simulink model "V2L"  (R2023a)
settings: Solver=ode23t  StartTime=0.0  StopTime=1  MaxStep=1e-4  RelTol=1e-3
undefined symbols (not defined in the file): Ion, Lithium
libraries: spsSeriesRLCBranchLib x5, spsCurrentMeasurementLib x2, spsVoltageMeasurementLib x2, spsBatteryLib x1, spsDiodeLib x1, spsMosfetLib x1, spsSeriesRLCLoadLib x1, slpidlib x1, spsPWMGenerator2LevelLib x1, spsPWMGeneratorDCDCLib x1, spsUniversalBridgeLib x1, spspowerguiLib x1
settings Model: Creator=Alielden  LastModifiedBy=Alielden

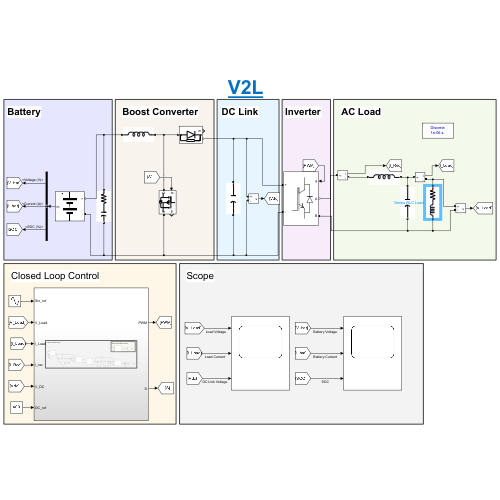
[thumbnail: Simulink's stored preview of the top-level diagram]
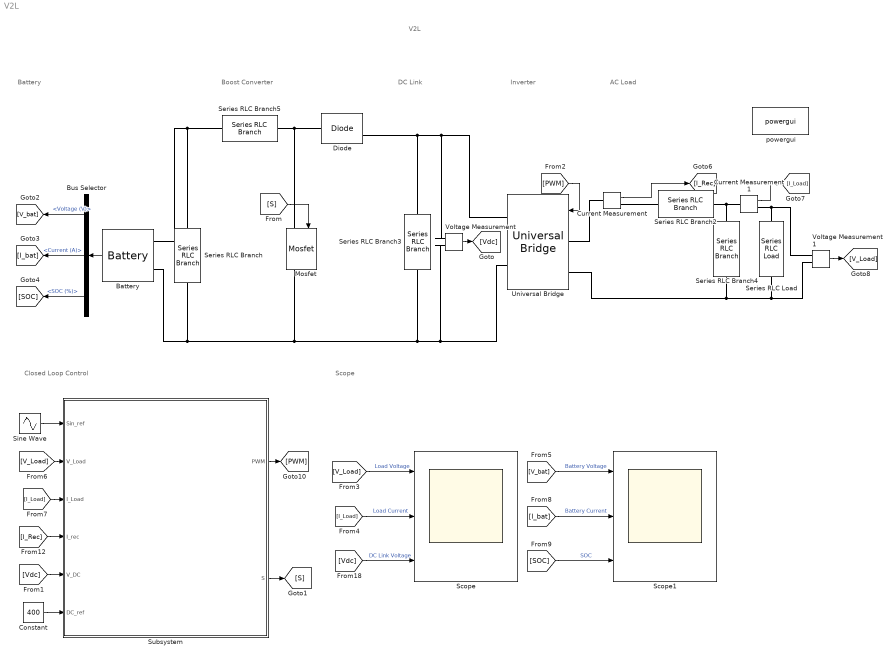
== system V2L ==
  note: Battery
  note: Boost Converter
  note: DC Link
  note: Inverter
  note: AC Load
  note: Closed Loop Control
  note: Scope
  note: V2L
  Battery : spsBatteryLib/Battery  BatType=Lithium-Ion  ShowTempParam=off  ThermalPreset=no  ShowAgeParam=off  NomV=160  NomQ=120  SOC=50  Batt_Tr=1  PresetModel=on  MaxQ=120  MinV=120  FullV=186.2379  Dis_rate=52.1739  R=0.013333  Normal_OP=108.5217  expZone="[172.8617      5.895652]"  current=[6.5 13 32.5]  Units=Time  Tci=20  NomT=20  T2=-30  MaxQ2=4.8  FullV2=7.1  Normal_OP2=5.655  expZone2="[6.58           1]"  Rca=0.6  ti=2000  Dp=0  Neq0=0  Tsim=1e6  Ta1=25  Qeol=5.4*0.9  Reol=0.013333*1.2  Char_age=[2.3478, 3]  Dis_age=[2.3478, 10]  N1=1500  N2=10500  N3=1000  N4=1400  Ta2=45  N5=950
  Bus Selector : BusSelector  OutputSignals=Voltage (V),Current (A),SOC (%)
  Constant : Constant  Value=400
  Current Measurement : spsCurrentMeasurementLib/Current Measurement  PhasorSimulation=off  OutputType=Complex  PSBequivalent=0
  Current Measurement1 : spsCurrentMeasurementLib/Current Measurement  PhasorSimulation=off  OutputType=Complex  PSBequivalent=0
  Diode : spsDiodeLib/Diode  Ron=0.001  Lon=0  Vf=0.8  IC=0  UseSnubber=0  Rs=500  Cs=250e-9  Measurements=on
  Mosfet : spsMosfetLib/Mosfet  Ron=0.1  Lon=0  Rd=0.01  Vfd=0  IC=0  Rs=1e5  Cs=inf  Measurements=on
  Scope : Scope  NumInputPorts=3
  Scope1 : Scope  NumInputPorts=3
  Series RLC Branch : spsSeriesRLCBranchLib/Series RLC Branch  LConnTagsString=__new0  RConnTagsString=__new0  BranchType=RC  Resistance=0.0001  Inductance=1e-3  SetiL0=off  InitialCurrent=0  Capacitance=100e-6  Setx0=off  InitialVoltage=0  Measurements=None
  Series RLC Branch2 : spsSeriesRLCBranchLib/Series RLC Branch  LConnTagsString=__new0  RConnTagsString=__new0  BranchType=L  Resistance=1  Inductance=2e-3  SetiL0=off  InitialCurrent=0  Capacitance=5600e-6  Setx0=off  InitialVoltage=400  Measurements=None
  Series RLC Branch3 : spsSeriesRLCBranchLib/Series RLC Branch  LConnTagsString=__new0  RConnTagsString=__new0  BranchType=C  Resistance=1  Inductance=1e-3  SetiL0=off  InitialCurrent=0  Capacitance=5600e-6  Setx0=on  InitialVoltage=400  Measurements=None
  Series RLC Branch4 : spsSeriesRLCBranchLib/Series RLC Branch  LConnTagsString=__new0  RConnTagsString=__new0  BranchType=C  Resistance=1  Inductance=2e-3  SetiL0=off  InitialCurrent=0  Capacitance=5e-6  Setx0=off  InitialVoltage=400  Measurements=None
  Series RLC Branch5 : spsSeriesRLCBranchLib/Series RLC Branch  LConnTagsString=__new0  RConnTagsString=__new0  BranchType=L  Resistance=0.0001  Inductance=20e-3  SetiL0=off  InitialCurrent=0  Capacitance=100e-6  Setx0=off  InitialVoltage=0  Measurements=None
  Series RLC Load : spsSeriesRLCLoadLib/Series RLC Load  LConnTagsString=a  RConnTagsString=__new0  NominalVoltage=220  NominalFrequency=50  ActivePower=3e3  InductivePower=2e3  CapacitivePower=0  Setx0=off  InitialVoltage=0  SetiL0=off  InitialCurrent=0  Measurements=None  LoadType=constant Z
  Sine Wave : Sin  Amplitude=310  Frequency=2*pi*50  SampleTime=0
  Subsystem : Subsystem
  Universal Bridge : spsUniversalBridgeLib/Universal Bridge  Arms=2  SnubberResistance=1e5  SnubberCapacitance=inf  Device=IGBT / Diodes  Ron=1e-3  Lon=0  ForwardVoltages="[  0  0  ]"  ForwardVoltage=0  GTOparameters=[ 10e-6 , 20e-6 ]  IGBTparameters=[ 1e-6 , 2e-6 ]  Measurements=None  Measurements_2=None  converterType=Rectifier
  Voltage Measurement : spsVoltageMeasurementLib/Voltage Measurement  PhasorSimulation=off  OutputType=Complex  PSBequivalent=0
  Voltage Measurement1 : spsVoltageMeasurementLib/Voltage Measurement  PhasorSimulation=off  OutputType=Complex  PSBequivalent=0
  powergui : spspowerguiLib/powergui  Priority=1  SimulationMode=Discrete  SampleTime=1e-6  frequency=60  Iterations=50  frequencyindice=0  Pbase=100e6  ErrMax=1e-4  UnitsV=kV  UnitsW=MW  buscounter=0  FunctionMessages=off  echomessages=off  EnableUseOfTLC=off  CurrentSourceSwitches=off  DisableSnubberDevices=off  DisableRonSwitches=off  DisableVfSwitches=off  DisplayEquations=off  AutomaticDiscreteSolvers=off  SolverType=Tustin/Backward Euler (TBE)  Interpol=off  ExternalGateDelay=off  methode=off  Ts=100  x0status=blocks  SPID=on  SwTol=0  HookPort=off  NonlinearTolerance=1e-4  nMaxIteration=100  ContinueOnMaxIteration=off  RestoreLinks=warning  ResistiveCurrentMeasurement=off  Frange=[0:2:500]  Ylog=off  Xlog=on  ShowGrid=off  save=off  variable=ZData  structure=0  ZoomFFT=off  StartTime=0.0  cycles=1  DisplayStyle=1  fundamental=60  FreqAxis=off  MaxFrequency=1000  frequencyindicesteady=1  RmsSteady=1  display=off
  wires:
  Voltage Measurement/1 -> [Vdc]
  Current Measurement/1 -> [I_Rec]
  Current Measurement1/1 -> [I_Load]
  Voltage Measurement1/1 -> [V_Load]
  [V_Load] -> Scope/1  "Load Voltage"
  [S] -> Mosfet/1
  [PWM] -> Universal Bridge/1
  Battery/1 -> Bus Selector/1
  Bus Selector/1 -> [V_bat]  "<Voltage (V)>"
  Bus Selector/2 -> [I_bat]  "<Current (A)>"
  Bus Selector/3 -> [SOC]  "<SOC (%)>"
  Sine Wave/1 -> Subsystem/1(Sin_ref)
  [V_Load] -> Subsystem/2(V_Load)
  [I_Load] -> Subsystem/3(I_Load)
  [I_Rec] -> Subsystem/4(I_rec)
  [Vdc] -> Subsystem/5(V_DC)
  Subsystem/1(PWM) -> [PWM]
  Constant/1 -> Subsystem/6(DC_ref)
  Subsystem/2(S) -> [S]
  [I_Load] -> Scope/2  "Load Current"
  [Vdc] -> Scope/3  "DC Link Voltage"
  [V_bat] -> Scope1/1  "Battery Voltage"
  [I_bat] -> Scope1/2  "Battery Current"
  [SOC] -> Scope1/3  "SOC"
  connections:
  Battery/LConn1 -- Series RLC Branch5/RConn1 -- Series RLC Branch/LConn1
  Series RLC Branch4/LConn1 -- Current Measurement1/LConn1 -- Series RLC Branch2/RConn1
  Current Measurement1/RConn1 -- Voltage Measurement1/LConn1 -- Series RLC Load/LConn1
  Diode/LConn1 -- Series RLC Branch5/LConn1 -- Mosfet/LConn1
  Universal Bridge/LConn1 -- Current Measurement/LConn1
  Battery/LConn2 -- Series RLC Branch/RConn1 -- Series RLC Branch3/RConn1 -- Voltage Measurement/LConn2 -- Universal Bridge/RConn2 -- Mosfet/RConn1
  Diode/RConn1 -- Series RLC Branch3/LConn1 -- Voltage Measurement/LConn1 -- Universal Bridge/RConn1
  Series RLC Branch2/LConn1 -- Current Measurement/RConn1
  Universal Bridge/LConn2 -- Series RLC Branch4/RConn1 -- Voltage Measurement1/LConn2 -- Series RLC Load/RConn1

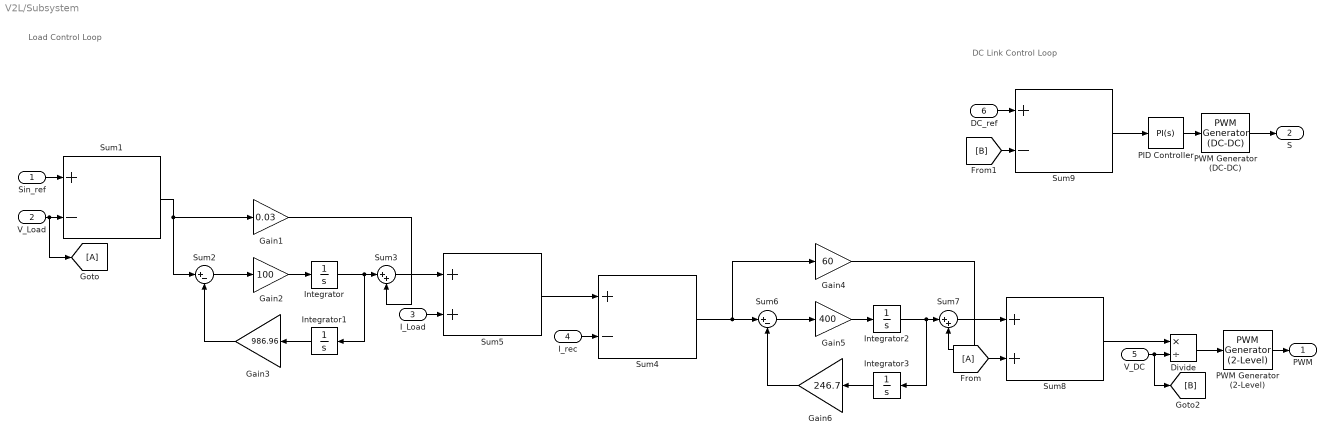
== system V2L/Subsystem ==
  note: Load Control Loop
  note: DC Link Control Loop
  Sin_ref : Inport
  V_Load : Inport  Port=2
  I_Load : Inport  Port=3
  I_rec : Inport  Port=4
  V_DC : Inport  Port=5
  DC_ref : Inport  Port=6
  Divide : Product  Inputs=*/
  From : From
  Gain1 : Gain  Gain=0.03
  Gain2 : Gain  Gain=100
  Gain3 : Gain  Gain=986.96
  Gain4 : Gain  Gain=60
  Gain5 : Gain  Gain=400
  Gain6 : Gain  Gain=246.7
  Goto : Goto
  Integrator{,1..3} (4 alike) : Integrator
  PID Controller : slpidlib/PID Controller  Controller=PI  Form=Parallel  TimeDomain=Continuous-time  UseExternalTs=off  SampleTime=-1  IntegratorMethod=Forward Euler  FilterMethod=Forward Euler  ControllerParametersSource=internal  P=0.005  I=0.05  UseKiTs=off  D=0  N=100  UseFilter=on  TunerSelectOption=Transfer Function Based (PID Tuner App)  InitialConditionSource=internal  InitialConditionForIntegrator=0  InitialConditionForFilter=0  DifferentiatorICPrevScaledInput=0  ExternalReset=none  TrackingMode=off  Kt=1  LimitOutput=on  SatLimitsSource=internal  UpperSaturationLimit=0.95  LowerSaturationLimit=0  LinearizeAsGain=on  AntiWindupMode=none  Kb=1  LimitIntegrator=off  UpperIntegratorSaturationLimit=inf  LowerIntegratorSaturationLimit=-inf  POutMin=[]  POutMax=[]  IOutMin=[]  IOutMax=[]  DOutMin=[]  DOutMax=[]  NOutMin=[]  NOutMax=[]  SumOutMin=[]  SumOutMax=[]  SaturationOutMin=[]  SaturationOutMax=[]  PParamMin=[]  PParamMax=[]  IParamMin=[]  IParamMax=[]  DParamMin=[]  DParamMax=[]  NParamMin=[]  NParamMax=[]  KbParamMin=[]  KbParamMax=[]  KtParamMin=[]  KtParamMax=[]  KbOutMin=[]  KbOutMax=[]  KtOutMin=[]  KtOutMax=[]  IntegratorOutMin=[]  IntegratorOutMax=[]  FilterOutMin=[]  FilterOutMax=[]  SumI1OutMin=[]  SumI1OutMax=[]  SumI2OutMin=[]  SumI2OutMax=[]  SumI3OutMin=[]  SumI3OutMax=[]  SumI4OutMin=[]  SumI4OutMax=[]  SumDOutMin=[]  SumDOutMax=[]  DifferentiatorOutMin=[]  DifferentiatorOutMax=[]  FilterDiffOutCoefMin=[]  FilterDiffOutCoefMax=[]  ReciprocalOutMin=[]  ReciprocalOutMax=[]  SumDenOutMin=[]  SumDenOutMax=[]  SumNumOutMin=[]  SumNumOutMax=[]  DivideOutMin=[]  DivideOutMax=[]  UdiffTsProdOutMin=[]  UdiffTsProdOutMax=[]  NTsProdOutMin=[]  NTsProdOutMax=[]  UintegralTsProdOutMin=[]  UintegralTsProdOutMax=[]  UngainTsProdOutMin=[]  UngainTsProdOutMax=[]  ClampingZeroOutDataTypeStr=Inherit: Inherit via back propagation  ClampingZeroOutMin=[]  ClampingZeroOutMax=[]  FilterDenConstantOutDataTypeStr=Inherit: Inherit via back propagation  FilterDenConstantOutMin=[]  FilterDenConstantOutMax=[]  PCopyOutDataTypeStr=Inherit: Inherit via back propagation  PCopyOutMin=[]  PCopyOutMax=[]  NCopyOutDataTypeStr=Inherit: Inherit via back propagation  NCopyOutMin=[]  NCopyOutMax=[]  IntegratorContinuousStateAttributes=''  IntegratorStateMustResolveToSignalObject=off  IntegratorRTWStateStorageClass=Auto  FilterContinuousStateAttributes=''  FilterStateMustResolveToSignalObject=off  FilterRTWStateStorageClass=Auto  ParallelPVariant=InternalParameters  IdealPVariant=Disabled  IVariant=InternalParameters  DVariant=Disabled  IntegratorVariant=Continuous  SatVariant=Enabled  AWVariant=Passthrough  PCopyVariant=Disabled  TRVariant=Disabled  FdbkBlocksVariant=Forward  IdealPFdbkVariant=Disabled  SatFdbkVariant=Disabled  DerivativeFilterVariant=Disabled  NVariant=Disabled  NCopyVariant=Disabled_SignalSpec  FilterICVariant=Disabled  IntegratorICVariant=InternalICs  ExternalResetVariant=Disabled  TRSumVariant=Passthrough  SumFdbkVariant=Disabled  SumVariant=Sum_PI  TsampFilterVariant=InternalTs  TsampNgainVariant=Passthrough  TsampIntegralVariant=Disabled_SignalSpec  ExternalSaturationOutDataTypeStr=Inherit: Same as second input
  PWM Generator (2-Level) : spsPWMGenerator2LevelLib/PWM Generator (2-Level)  ModulatorType=Single-phase full-bridge (4 pulses)  ModulatorMode=Unsynchronized  Fc=10000  Pc=90  nF=27  MinMax="[ -1  1 ]"  SamplingTechnique=Natural  ModulatingSignals=off  m=0.8  Freq=60  Phase=0  Ts=0  ShowCarrierOutport=off
  PWM Generator (DC-DC) : spsPWMGeneratorDCDCLib/PWM Generator (DC-DC)  Fsw=10000  Ts=0
  Sum1 : Sum  Inputs=+-
  Sum2 : Sum  Inputs=|+-
  Sum3 : Sum  Inputs=|++
  Sum4 : Sum  Inputs=+-
  Sum5 : Sum
  Sum6 : Sum  Inputs=|+-
  Sum7 : Sum  Inputs=|++
  Sum8 : Sum
  Sum9 : Sum  Inputs=+-
  PWM : Outport
  S : Outport  Port=2
  wires:
  Sum4/1 -> Gain4/1, Sum6/1
  Gain4/1 -> Sum7/2
  Integrator1/1 -> Gain3/1
  Integrator/1 -> Integrator1/1, Sum3/1
  Sum2/1 -> Gain2/1
  Gain5/1 -> Integrator2/1
  Gain1/1 -> Sum3/2
  Integrator2/1 -> Integrator3/1, Sum7/1
  Integrator3/1 -> Gain6/1
  Gain3/1 -> Sum2/2
  Sum3/1 -> Sum5/1
  Sum8/1 -> Divide/1
  Sum7/1 -> Sum8/1
  Sum6/1 -> Gain5/1
  Sum1/1 -> Sum2/1, Gain1/1
  Sum5/1 -> Sum4/1
  Gain2/1 -> Integrator/1
  Gain6/1 -> Sum6/2
  Sin_ref/1 -> Sum1/1
  V_Load/1 -> Goto/1, Sum1/2
  I_Load/1 -> Sum5/2
  I_rec/1 -> Sum4/2
  From/1 -> Sum8/2
  V_DC/1 -> [B], Divide/2
  Divide/1 -> PWM Generator (2-Level)/1
  PWM Generator (2-Level)/1 -> PWM/1
  PID Controller/1 -> PWM Generator (DC-DC)/1
  Sum9/1 -> PID Controller/1
  PWM Generator (DC-DC)/1 -> S/1
  DC_ref/1 -> Sum9/1
  [B] -> Sum9/2
